simulink model "Book7242"  (R2019b)
settings: Solver=ode4  StartTime=0.0  StopTime=10.0  FixedStep=0.001  RelTol=1e-3
libraries: fuzblock x2
settings Model: Creator=user  LastModifiedBy=xyh

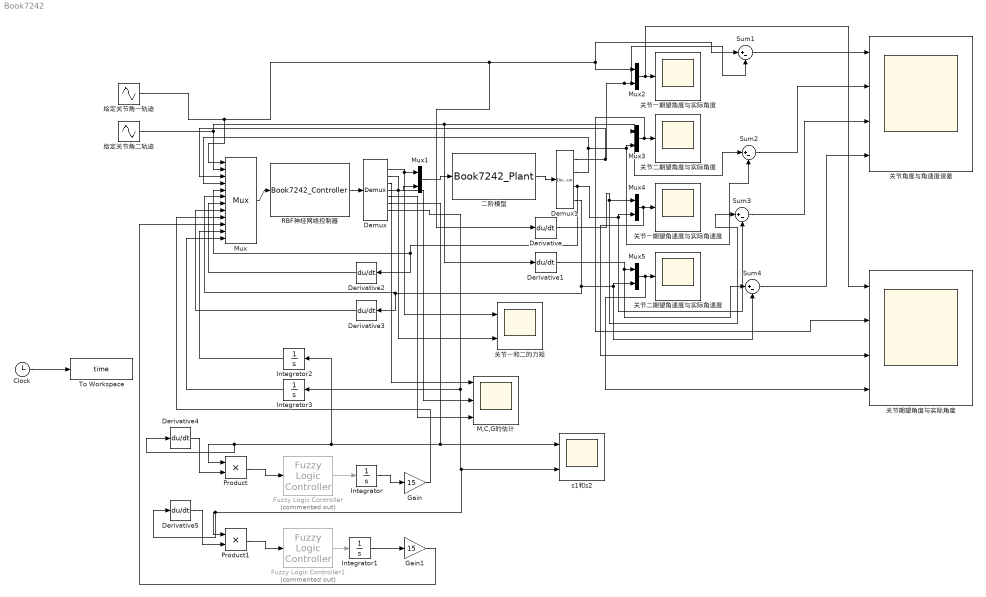
== system Book7242 ==
  Clock : Clock
  Demux : Demux  Outputs=7
  Demux1 : Demux
  Derivative{,1..5} (6 alike) : Derivative
  Fuzzy Logic Controller : fuzblock/Fuzzy Logic  Controller  Commented=on  FIS=Book434  OutputSampleNumber=101  DataType=double  FuzzifiedInputs=off  RuleFiringStrengths=off  RuleOutputs=off  AggregatedOutputs=off  SimulateUsing=Interpreted execution  OutOfRangeInputValueMessage=warning  NoRuleFiredMessage=warning  EmptyOutputFuzzySetMessage=warning
  Fuzzy Logic Controller1 : fuzblock/Fuzzy Logic  Controller  Commented=on  FIS=Book434  OutputSampleNumber=101  DataType=double  FuzzifiedInputs=off  RuleFiringStrengths=off  RuleOutputs=off  AggregatedOutputs=off  SimulateUsing=Interpreted execution  OutOfRangeInputValueMessage=warning  NoRuleFiredMessage=warning  EmptyOutputFuzzySetMessage=warning
  Gain : Gain  Gain=15
  Gain1 : Gain  Gain=15
  Integrator{,1..3} (4 alike) : Integrator
  M,C,G的估计 : Scope  NumInputPorts=3
  Mux : Mux  Inputs=12
  Mux{1..5} (5 alike) : Mux  Inputs=2
  Product : Product
  Product1 : Product
  RBF神经网络控制器 : S-Function  FunctionName=Book7242_Controller  SFunctionDeploymentMode=off  EnableBusSupport=off
  Sum{1..4} (4 alike) : Sum  Inputs=|+-
  To Workspace : ToWorkspace  VariableName=time  SaveFormat=Timeseries  SampleTime=-1
  s1和s2 : Scope  NumInputPorts=2
  二阶模型 : S-Function  FunctionName=Book7242_Plant  SFunctionDeploymentMode=off  EnableBusSupport=off
  关节一和二的力矩 : Scope  NumInputPorts=2
  关节一期望角度与实际角度 : Scope
  关节一期望角速度与实际角速度 : Scope
  关节二期望角度与实际角度 : Scope
  关节二期望角速度与实际角速度 : Scope
  关节期望角度与实际角度 : Scope  NumInputPorts=4
  关节角度与角速度误差 : Scope  NumInputPorts=4
  给定关节角一轨迹 : Sin  Amplitude=0.5  Frequency=pi  SampleTime=0
  给定关节角二轨迹 : Sin  Amplitude=0.5  Frequency=pi  SampleTime=0
  wires:
  二阶模型/1 -> Demux1/1
  Derivative/1 -> Mux4/1, Sum3/1
  Derivative1/1 -> Mux5/1, Sum4/1
  Mux/1 -> RBF神经网络控制器/1
  Mux1/1 -> 二阶模型/1
  给定关节角二轨迹/1 -> Mux/2, Mux3/1, Sum2/1, Derivative1/1
  Demux1/1 -> Mux/3, Sum1/2, Mux2/2
  Clock/1 -> To Workspace/1
  Demux/2 -> 关节一和二的力矩/2, Mux1/2
  Demux/1 -> Mux1/1, 关节一和二的力矩/1
  Derivative2/1 -> Mux/7
  Demux1/3 -> Derivative2/1, Mux/5, Mux4/2, Sum3/2
  Demux1/4 -> Mux5/2, Sum4/2, Derivative3/1, Mux/6
  给定关节角一轨迹/1 -> Derivative/1, Mux2/1, Sum1/1, Mux/1
  Demux1/2 -> Mux/4, Mux3/2, Sum2/2
  RBF神经网络控制器/1 -> Demux/1
  Derivative3/1 -> Mux/8
  Demux/3 -> M,C,G的估计/1
  Demux/4 -> M,C,G的估计/2
  Demux/5 -> M,C,G的估计/3
  Sum2/1 -> 关节角度与角速度误差/2
  Sum1/1 -> 关节角度与角速度误差/1
  Sum4/1 -> 关节角度与角速度误差/4
  Sum3/1 -> 关节角度与角速度误差/3
  Demux/6 -> s1和s2/1, Integrator2/1, Derivative4/1, Product/1
  Demux/7 -> Derivative5/1, Product1/1, s1和s2/2, Integrator3/1
  Mux2/1 -> 关节期望角度与实际角度/1, 关节一期望角度与实际角度/1
  Mux3/1 -> 关节期望角度与实际角度/2, 关节二期望角度与实际角度/1
  Mux4/1 -> 关节期望角度与实际角度/3, 关节一期望角速度与实际角速度/1
  Mux5/1 -> 关节期望角度与实际角度/4, 关节二期望角速度与实际角速度/1
  Derivative4/1 -> Product/2
  Product/1 -> Fuzzy Logic Controller/1
  Fuzzy Logic Controller/1 -> Integrator/1
  Derivative5/1 -> Product1/2
  Product1/1 -> Fuzzy Logic Controller1/1
  Integrator/1 -> Gain/1
  Integrator1/1 -> Gain1/1
  Gain/1 -> Mux/9
  Gain1/1 -> Mux/10
  Fuzzy Logic Controller1/1 -> Integrator1/1
  Integrator2/1 -> Mux/11
  Integrator3/1 -> Mux/12
